simulink model "Final_System_Model"  (R2018a)
settings: Solver=VariableStepAuto  StartTime=0  StopTime=inf  RelTol=1e-3
PreLoadFcn:
  | Ts_Power=1e-6;
  | Ts_Control=100e-6;
undefined symbols (not defined in the file): DiscIntNeverNeededParam, FC, FuelCellLoadFcn, gcbh, Ion, Lithium, sigbuilder_block, sps_rtmsupport
libraries: powerlib x13, simulink x8, fl_lib x8, nesl_utility x6, powerlib_meascontrol x5, electricdrivelib x1, spsFuelCellModel x1, re_lib x1
(part 4 of 4)

== system Final_System_Model/Electrolyzer Stack/electrolyser stack/electrolyser cell/eta_c/m_c ==
  In1 : Inport
  Constant : Constant
  Divide : Product  Inputs=*/
  Subtract : Sum  Inputs=+-
  limiting current : Constant  Value=0.00023
  Out1 : Outport
  wires:
  Constant/1 -> Subtract/1
  Subtract/1 -> Out1/1
  limiting current/1 -> Divide/2
  Divide/1 -> Subtract/2
  In1/1 -> Divide/1

== system Final_System_Model/Electrolyzer Stack/electrolyser stack/electrolyser cell/eta_c/n_c ==
  In1 : Inport
  In2 : Inport  Port=2
  In3 : Inport  Port=3
  Divide : Product  Inputs=*/
  i_c0 : Subsystem
  Out1 : Outport
  wires:
  In2/1 -> i_c0/1(In1)
  i_c0/1(Out1) -> Divide/2
  In1/1 -> i_c0/2(In2)
  Divide/1 -> Out1/1
  In3/1 -> Divide/1

== system Final_System_Model/Fuel Cell Stack/Fuel Cell Model/ From Current Density (A//cm^2) To Overvoltages (V)/Concentration Overvoltage/IF Function ==
  In1 : Inport
  Compare To Zero : simulink/Logic and Bit Operations/Compare To Zero  relop=<=  OutDataTypeStr=boolean
  If : If  IfExpression=u1 == 0
  If Action Subsystem : Subsystem  TreatAsAtomicUnit=on
  If Action Subsystem1 : Subsystem  TreatAsAtomicUnit=on
  Merge : Merge  InitialOutput=1
  Out1 : Outport
  wires:
  If Action Subsystem1/1(Out1) -> Merge/2
  Compare To Zero/1 -> If/1
  Merge/1 -> Out1/1
  In1/1 -> If Action Subsystem/1(In1), Compare To Zero/1
  If/2 -> If Action Subsystem1/Action
  If Action Subsystem/1(Out1) -> Merge/1
  If/1 -> If Action Subsystem/Action

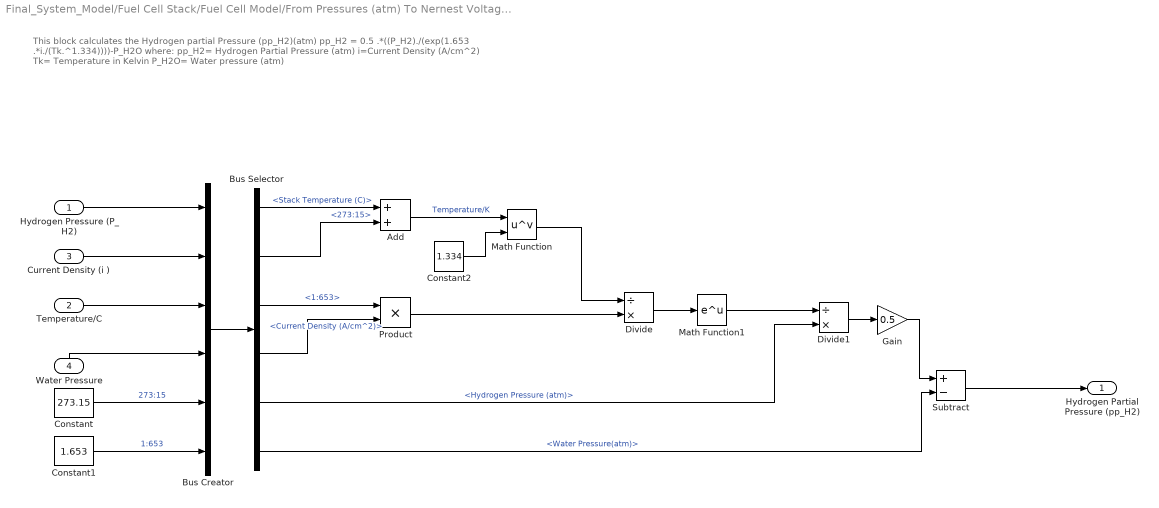
== system Final_System_Model/Fuel Cell Stack/Fuel Cell Model/From Pressures (atm) To Nernest Voltage (V)/From Absolute Pressure (atm) To Partial Pressures (atm)/Hydrogen Partial Pressure Output ==
  note: This block calculates the Hydrogen partial Pressure (pp_H2)(atm)
      | pp_H2 = 0.5 .*((P_H2)./(exp(1.653 .*i./(Tk.^1.334))))-P_H2O
      | where: pp_H2= Hydrogen Partial Pressure (atm)
      | i=Current Density (A/cm^2)
      | Tk= Temperature in Kelvin
      | P_H2O= Water pressure (atm)
  Hydrogen Pressure (P_H2) : Inport
  Temperature/C : Inport  Port=2
  Current Density (i ) : Inport  Port=3
  Water Pressure : Inport  Port=4
  Add : Sum
  Bus Creator : BusCreator  Inputs=6
  Bus Selector : BusSelector  OutputSignals=Stack Temperature (C),273:15,1:653,Current Density (A/cm^2),Hydrogen Pressure (atm),Water Pressure(atm)
  Constant : Constant  Value=273.15
  Constant1 : Constant  Value=1.653
  Constant2 : Constant  Value=1.334
  Divide : Product  Inputs=/*
  Divide1 : Product  Inputs=/*
  Gain : Gain  Gain=0.5
  Math Function : Math  Operator=pow  SaturateOnIntegerOverflow=on
  Math Function1 : Math  SaturateOnIntegerOverflow=on
  Product : Product
  Subtract : Sum  Inputs=+-
  Hydrogen Partial Pressure (pp_H2) : Outport
  wires:
  Water Pressure/1 -> Bus Creator/4
  Temperature/C/1 -> Bus Creator/3
  Current Density (i )/1 -> Bus Creator/2
  Hydrogen Pressure (P_H2)/1 -> Bus Creator/1
  Bus Creator/1 -> Bus Selector/1
  Bus Selector/5 -> Divide1/2  "<Hydrogen Pressure (atm)>"
  Bus Selector/1 -> Add/1  "<Stack Temperature (C)>"
  Constant/1 -> Bus Creator/5  "273:15"
  Add/1 -> Math Function/1  "Temperature/K"
  Constant1/1 -> Bus Creator/6  "1:653"
  Bus Selector/2 -> Add/2  "<273:15>"
  Bus Selector/3 -> Product/1  "<1:653>"
  Bus Selector/4 -> Product/2  "<Current Density (A/cm^2)>"
  Product/1 -> Divide/2
  Divide/1 -> Math Function1/1
  Constant2/1 -> Math Function/2
  Math Function/1 -> Divide/1
  Math Function1/1 -> Divide1/1
  Divide1/1 -> Gain/1
  Bus Selector/6 -> Subtract/2  "<Water Pressure(atm)>"
  Subtract/1 -> Hydrogen Partial Pressure (pp_H2)/1
  Gain/1 -> Subtract/1

== system Final_System_Model/Fuel Cell Stack/Fuel Cell Model/From Pressures (atm) To Nernest Voltage (V)/From Absolute Pressure (atm) To Partial Pressures (atm)/Oxygen Partial Pressure Output ==
  note: This block calculates the Oxygen Partial Pressure (atm)
      | pp_O2 = (P_air./exp(4.192 .*i/(Tk.^1.334)))-P_H2O
      |
      | where: pp_O2= Oxygen Partial Pressure (atm)
      | P_air= Air Pressure (atm)
      | i= Current Density (A/cm^2)
      | Tk= Temperature (K)
      | P_H2O=Water Pressure (atm)
  Air Pressure (P_air) : Inport
  Temperature/C : Inport  Port=2
  Current Density/i : Inport  Port=3
  Water Pressure : Inport  Port=4
  Add : Sum
  Bus Creator : BusCreator  Inputs=7
  Bus Selector : BusSelector  OutputSignals=Stack Temperature (C),273:15,1:334,Current Density (A/cm^2),4:192,Air Pressure (atm),Water Pressure(atm)
  Constant : Constant  Value=273.15
  Constant1 : Constant  Value=4.192
  Constant2 : Constant  Value=1.334
  Divide : Product  Inputs=/*
  Divide1 : Product  Inputs=/*
  Math Function : Math  Operator=pow  SaturateOnIntegerOverflow=on
  Math Function1 : Math  SaturateOnIntegerOverflow=on
  Product : Product
  Subtract : Sum  Inputs=+-
  Oxygen Partial Pressure pp_O2 : Outport
  wires:
  Current Density/i/1 -> Bus Creator/2
  Water Pressure/1 -> Bus Creator/4
  Temperature/C/1 -> Bus Creator/3
  Air Pressure (P_air)/1 -> Bus Creator/1
  Constant/1 -> Bus Creator/5  "273:15"
  Constant1/1 -> Bus Creator/6  "4:192"
  Constant2/1 -> Bus Creator/7  "1:334"
  Bus Creator/1 -> Bus Selector/1
  Bus Selector/1 -> Add/1  "<Stack Temperature (C)>"
  Bus Selector/2 -> Add/2  "<273:15>"
  Add/1 -> Math Function/1  "Temperature/K"
  Bus Selector/3 -> Math Function/2  "<1:334>"
  Bus Selector/4 -> Product/1  "<Current Density (A/cm^2)>"
  Bus Selector/5 -> Product/2  "<4:192>"
  Product/1 -> Divide/2
  Math Function/1 -> Divide/1
  Divide/1 -> Math Function1/1
  Math Function1/1 -> Divide1/1
  Bus Selector/6 -> Divide1/2  "<Air Pressure (atm)>"
  Divide1/1 -> Subtract/1
  Bus Selector/7 -> Subtract/2  "<Water Pressure(atm)>"
  Subtract/1 -> Oxygen Partial Pressure pp_O2/1  "Oxygen Partial Pressure pp_O2 (atm)"

== system Final_System_Model/Fuel Cell Stack/Fuel Cell Model/From Pressures (atm) To Nernest Voltage (V)/From Absolute Pressure (atm) To Partial Pressures (atm)/Water Pressure output ==
  note: This block calculates the water saturation Pressure (atm) from the Fuel Cell Temperature (k)
      | x = -2.1794 + 0.02953 .*Tc-9.1837 .*(10.^-5) .*(Tc.^2) + 1.4454 .*(10.^-7) .*(Tc.^3);
      | where: x=Water Saturation Pressure (atm)
      | Tc= Temperature in degree celsius
  Temperature/C : Inport
  -1 : Constant  Value=-7
  -2 : Constant  Value=3
  -5 : Constant  Value=-5
  0.02953 : Constant  Value=0.02953
  0.1 : Constant  Value=9.1837
  0.2 : Constant  Value=1.4454
  Add : Sum  Inputs=+++-
  Constant4 : Constant  Value=-2.1794
  Math Function4 : Math  Operator=10^u  SaturateOnIntegerOverflow=on
  Math Function5 : Math  Operator=square  SaturateOnIntegerOverflow=on
  Math Function6 : Math  Operator=10^u  SaturateOnIntegerOverflow=on
  Math Function7 : Math  Operator=pow  SaturateOnIntegerOverflow=on
  Product1 : Product  Inputs=3
  Product2 : Product
  Product3 : Product  Inputs=3
  "water  pressure " : Math  Operator=10^u  SaturateOnIntegerOverflow=on
  Water Pressure : Outport
  wires:
  Add/1 -> "water  pressure "/1
  0.2/1 -> Product3/1
  Math Function7/1 -> Product3/3
  "water  pressure "/1 -> Water Pressure/1  "Water Pressure(atm)"
  0.02953/1 -> Product2/1
  0.1/1 -> Product1/1
  -5/1 -> Math Function4/1
  Math Function4/1 -> Product1/2
  -1/1 -> Math Function6/1
  Temperature/C/1 -> Product2/2, Math Function5/1, Math Function7/1
  Math Function5/1 -> Product1/3
  -2/1 -> Math Function7/2
  Product2/1 -> Add/2
  Product3/1 -> Add/3
  Math Function6/1 -> Product3/2
  Constant4/1 -> Add/1
  Product1/1 -> Add/4

== system Final_System_Model/Fuel Cell Stack/Fuel Cell Model/From Pressures (atm) To Nernest Voltage (V)/From Partial Pressures (atm) To Nernest Voltage (V)/IF Function ==
  In1 : Inport
  Constant1 : Constant
  If : If
  If Action Subsystem : Subsystem  TreatAsAtomicUnit=on
  If Action Subsystem1 : Subsystem  TreatAsAtomicUnit=on
  Merge : Merge
  Out1 : Outport
  wires:
  Constant1/1 -> If Action Subsystem1/1(In1)
  If Action Subsystem1/1(Out1) -> Merge/2
  If/1 -> If Action Subsystem/Action
  If/2 -> If Action Subsystem1/Action
  In1/1 -> If Action Subsystem/1(In1), If/1
  Merge/1 -> Out1/1
  If Action Subsystem/1(Out1) -> Merge/1

== system Final_System_Model/Electrolyzer Stack/electrolyser stack/electrolyser cell/Eta_B/segma_B/Beta ==
  In1 : Inport
  In2 : Inport  Port=2
  Add3 : Sum
  Add4 : Sum  Inputs=-+
  Add5 : Sum  Inputs=+-
  Add6 : Sum  Inputs=-+
  Constant3 : Constant
  Constant4 : Constant  Value=4
  Constant5 : Constant  Value=2
  Math Function1 : Math  Operator=square  SaturateOnIntegerOverflow=on
  Product5 : Product  Inputs=***
  Product6 : Product  Inputs=*/
  Product7 : Product  Inputs=*/
  Product8 : Product  Inputs=**
  Sqrt : Sqrt  SaturateOnIntegerOverflow=on
  Out1 : Outport
  wires:
  Math Function1/1 -> Add4/2
  Constant3/1 -> Product6/1, Add5/1, Add3/1
  Add3/1 -> Add6/2, Math Function1/1
  Sqrt/1 -> Add6/1
  Constant4/1 -> Product5/1
  Constant5/1 -> Product8/2
  Add4/1 -> Sqrt/1
  Product6/1 -> Add5/2
  Product5/1 -> Add4/1
  Add6/1 -> Product7/1
  Product8/1 -> Product7/2
  Product7/1 -> Out1/1
  In1/1 -> Product5/2, Add3/2
  In2/1 -> Product6/2
  Add5/1 -> Product8/1, Product5/3

== system Final_System_Model/Electrolyzer Stack/electrolyser stack/electrolyser cell/Eta_B/segma_B/K_a ==
  In1 : Inport
  In2 : Inport  Port=2
  In3 : Inport  Port=3
  Add2 : Sum  Inputs=+-
  Constant : Constant  Value=-523000
  Constant1 : Constant
  Math Function : Math  SaturateOnIntegerOverflow=on
  Product2 : Product  Inputs=*/
  Product3 : Product  Inputs=*/
  Product4 : Product
  Out1 : Outport
  Out2 : Outport  Port=2
  wires:
  Product4/1 -> Math Function/1
  Add2/1 -> Out2/1, Product4/2
  Math Function/1 -> Out1/1
  In3/1 -> Add2/2
  In2/1 -> Product3/2
  Product2/1 -> Product4/1
  Constant1/1 -> Product3/1
  Product3/1 -> Add2/1
  Constant/1 -> Product2/1
  In1/1 -> Product2/2

== system Final_System_Model/Electrolyzer Stack/electrolyser stack/electrolyser cell/Eta_B/segma_B/eta_B ==
  In1 : Inport
  In2 : Inport  Port=2
  Add : Sum
  Product : Product  Inputs=*/
  Out1 : Outport
  wires:
  Product/1 -> Out1/1
  In2/1 -> Add/2
  In1/1 -> Product/1, Add/1
  Add/1 -> Product/2

== system Final_System_Model/Electrolyzer Stack/electrolyser stack/electrolyser cell/Eta_B/segma_B/eta_B0 ==
  In1 : Inport
  In2 : Inport  Port=2
  Add1 : Sum
  Product1 : Product  Inputs=/*
  Out1 : Outport
  wires:
  Add1/1 -> Product1/1
  Product1/1 -> Out1/1
  In1/1 -> Add1/1
  In2/1 -> Product1/2, Add1/2

== system Final_System_Model/Electrolyzer Stack/electrolyser stack/electrolyser cell/eta_a/n_a/i_a0 ==
  In1 : Inport
  In2 : Inport  Port=2
  Divide : Product  Inputs=*/
  E_a : Constant  Value=76
  Exp : Math  SaturateOnIntegerOverflow=on
  Gain : Gain  Gain=-1
  Multiply : Product
  Multiply1 : Product  Inputs=3
  i_a0ref : Constant  Value=5e-12
  lamda_ma : Subsystem
  Out1 : Outport
  wires:
  Gain/1 -> Exp/1
  Exp/1 -> Multiply1/3
  Multiply/1 -> Gain/1
  Divide/1 -> Multiply/1
  i_a0ref/1 -> Multiply1/1
  In2/1 -> Multiply/2
  Multiply1/1 -> Out1/1
  E_a/1 -> Divide/1
  lamda_ma/1(Out1) -> Multiply1/2
  In1/1 -> Divide/2

== system Final_System_Model/Electrolyzer Stack/electrolyser stack/electrolyser cell/eta_c/n_c/i_c0 ==
  In1 : Inport
  In2 : Inport  Port=2
  Divide : Product  Inputs=*/
  E_c : Constant  Value=4.3
  Exp : Math  SaturateOnIntegerOverflow=on
  Gain : Gain  Gain=-1
  Multiply : Product  Inputs=3
  Multiply1 : Product
  i_c0ref : Constant  Value=1e-3
  lamda_mc : Subsystem
  Out1 : Outport
  wires:
  i_c0ref/1 -> Multiply/2
  Multiply/1 -> Out1/1
  Divide/1 -> Multiply1/2
  Multiply1/1 -> Gain/1
  E_c/1 -> Divide/1
  In1/1 -> Divide/2
  lamda_mc/1(Out1) -> Multiply/1
  Exp/1 -> Multiply/3
  Gain/1 -> Exp/1
  In2/1 -> Multiply1/1

== system Final_System_Model/Fuel Cell Stack/Fuel Cell Model/ From Current Density (A//cm^2) To Overvoltages (V)/Concentration Overvoltage/IF Function/If Action Subsystem ==
  In1 : Inport
  Action Port : ActionPort  ActionType=then
  Math Function1 : Math  Operator=log  OutputSignalType=real  SaturateOnIntegerOverflow=on
  Out1 : Outport
  wires:
  In1/1 -> Math Function1/1
  Math Function1/1 -> Out1/1

== system Final_System_Model/Fuel Cell Stack/Fuel Cell Model/ From Current Density (A//cm^2) To Overvoltages (V)/Concentration Overvoltage/IF Function/If Action Subsystem1 ==
  Action Port : ActionPort  ActionType=else
  Constant1 : Constant  Value=0
  Out1 : Outport
  wires:
  Constant1/1 -> Out1/1

== system Final_System_Model/Fuel Cell Stack/Fuel Cell Model/From Pressures (atm) To Nernest Voltage (V)/From Partial Pressures (atm) To Nernest Voltage (V)/IF Function/If Action Subsystem ==
  In1 : Inport
  Action Port : ActionPort  ActionType=then
  Out1 : Outport
  wires:
  In1/1 -> Out1/1

== system Final_System_Model/Fuel Cell Stack/Fuel Cell Model/From Pressures (atm) To Nernest Voltage (V)/From Partial Pressures (atm) To Nernest Voltage (V)/IF Function/If Action Subsystem1 ==
  In1 : Inport
  Action Port : ActionPort  ActionType=else
  Out1 : Outport
  wires:
  In1/1 -> Out1/1

== system Final_System_Model/Electrolyzer Stack/electrolyser stack/electrolyser cell/eta_a/n_a/i_a0/lamda_ma ==
  Constant : Constant  Value=6
  Divide : Product  Inputs=*/
  Gain : Gain  Gain=0.75
  Product : Product
  Product1 : Product
  d_ma : Constant  Value=2.9
  m_Ma : Constant  Value=1e-3
  rho_ma : Constant  Value=22.56
  Out1 : Outport
  wires:
  Gain/1 -> Product1/1
  Divide/1 -> Product1/2
  m_Ma/1 -> Gain/1
  d_ma/1 -> Product/2
  rho_ma/1 -> Product/1
  Product/1 -> Divide/2
  Constant/1 -> Divide/1
  Product1/1 -> Out1/1

== system Final_System_Model/Electrolyzer Stack/electrolyser stack/electrolyser cell/eta_c/n_c/i_c0/lamda_mc ==
  Constant : Constant  Value=6
  Divide : Product  Inputs=*/
  Gain : Gain  Gain=0.75
  Multiply : Product
  Multiply1 : Product
  d_mc : Constant  Value=2.7
  m_Mc : Constant  Value=0.3e-3
  rho_mc : Constant  Value=21.45
  Out1 : Outport
  wires:
  Gain/1 -> Multiply1/1
  Divide/1 -> Multiply1/2
  m_Mc/1 -> Gain/1
  Constant/1 -> Divide/1
  d_mc/1 -> Multiply/2
  Multiply/1 -> Divide/2
  Multiply1/1 -> Out1/1
  rho_mc/1 -> Multiply/1
